simulink model "StdAnimation_Test"  (R2017b)
settings: Solver=FixedStepDiscrete  StartTime=0.0  StopTime=45  FixedStep=0.02  RelTol=1e-3  EnableMultiTasking=on
undefined symbols (not defined in the file): sigbuilder_block
settings Model: DataDictionary=Copy_of_StdAnimation_DD_New.sldd  Creator=mchawa  LastModifiedBy=oashraf
settings ConfigSet: Description=AutoGeneratedSLSFconfig
settings DataIOCC: LimitDataPoints=on  SaveOutput=off  SaveTime=off
settings OptimizationCC: DefaultParameterBehavior=Inlined  UseDivisionForNetSlopeComputation=on  DefaultUnderspecifiedDataType=single  PassReuseOutputArgsAs=Individual arguments  LifeSpan=Inf  SimCompilerOptimization=on
settings DebuggingCC: ConsistencyChecking=warning  SignalInfNanChecking=error  SignalRangeChecking=error  ReadBeforeWriteMsg=EnableAllAsError  WriteAfterWriteMsg=EnableAllAsError  WriteAfterReadMsg=EnableAllAsError  AlgebraicLoopMsg=error  ArtificialAlgebraicLoopMsg=error  SaveWithDisabledLinksMsg=error  SaveWithParameterizedLinksMsg=error  SignalResolutionControl=TryResolveAllWithWarning  BlockPriorityViolationMsg=error  MinStepSizeMsg=error  SolverPrmCheckMsg=error  InheritedTsInSrcMsg=error  SingleTaskRateTransMsg=error  TasksWithSamePriorityMsg=error  SigSpecEnsureSampleTimeMsg=error  CheckMatrixSingularityMsg=error  ParameterDowncastMsg=warning  ParameterUnderflowMsg=error  FixptConstUnderflowMsg=warning  FixptConstOverflowMsg=warning  FixptConstPrecisionLossMsg=warning  UnderSpecifiedDataTypeMsg=warning  UnnecessaryDatatypeConvMsg=warning  VectorMatrixConversionMsg=warning  SignalLabelMismatchMsg=warning  UnconnectedInputMsg=error  UnconnectedOutputMsg=error  UnconnectedLineMsg=error  SFcnCompatibilityMsg=warning  FrameProcessingCompatibilityMsg=warning  UniqueDataStoreMsg=error  BusObjectLabelMismatch=none  RootOutportRequireBusObject=error  AssertControl=DisableAll  AllowSymbolicDim=off  ModelReferenceVersionMismatchMessage=warning  ModelReferenceIOMismatchMessage=warning  UnknownTsInhSupMsg=error  ModelReferenceDataLoggingMessage=error  StateNameClashWarn=warning  StrictBusMsg=ErrorOnBusTreatedAsVector  NonBusSignalsTreatedAsBus=error  SFInvalidInputDataAccessInChartInitDiag=error  SFTransitionOutsideNaturalParentDiag=error  SFUnreachableExecutionPathDiag=error  SFUndirectedBroadcastEventsDiag=error  SFTransitionActionBeforeConditionDiag=error  SFTemporalDelaySmallerThanSampleTimeDiag=error  SFSelfTransitionDiag=error  SFMachineParentedDataDiag=error
settings HardwareCC: ProdBitPerPointer=32  ProdBitPerSizeT=32  ProdBitPerPtrDiffT=32  ProdLargestAtomicInteger=Long  ProdLargestAtomicFloat=Double  ProdWordSize=32  ProdLongLongMode=on  ProdHWDeviceType=NXP->Cortex-M0/M0+
settings ModelReferenceCC: EnableRefExpFcnMdlSchedulingChecks=off  ModelReferenceNumInstancesAllowed=Single  PropagateSignalLabelsOutOfModel=off
settings SFSimCC: SimUserSources="\"ANIM_int.c\""  MATLABDynamicMemAlloc=off
settings RTWCC: SystemTargetFile=ert.tlc  TemplateMakefile=ert_default_tmf  BuildConfiguration=Faster Runs  IncludeHyperlinkInReport=on  PortableWordSizes=on  CodeExecutionProfiling=on  CodeProfilingInstrumentation=on
settings RTWCC: CustomSource=|
  | "ANIM_int.c"
  | "ANIM_cfg.c"
settings CodeAppCC: IgnoreCustomStorageClasses=off  IgnoreTestpoints=on  SimulinkDataObjDesc=on  SFDataObjDesc=on  CustomSymbolStrType=$N$R$M  CustomSymbolStrFcn=$N$M$F  CustomSymbolStrBlkIO=loc_$N$M  CustomSymbolStrTmpVar=loc_$N$M  InsertBlockDesc=on  StateflowObjectComments=on  ReqsInCode=on
settings ERTTargetCC: UtilityFuncGeneration=Shared location  GenerateSampleERTMain=on  IncludeMdlTerminateFcn=off  CombineSignalStateStructs=on  SuppressErrorStatus=on  SupportAbsoluteTime=off  SupportNonFinite=off  SupportComplex=off  PurelyIntegerCode=on  RemoveResetFunc=off  ParenthesesLevel=Maximum  CastingMode=Standards  GenerateSharedConstants=off  GenerateASAP2=on  ERTCustomFileTemplate=example_file_process.tlc  EnableDataOwnership=on  DataDefinitionFile=ADBM_cfg.c  DataReferenceFile=ADBM_cfg.h  ConvertIfToSwitch=off  SuppressUnreachableDefaultCases=off  EnableSignedLeftShifts=off  EnableSignedRightShifts=off  MemSecPackage=mpt
settings ConfigComp: CovMetricSettings=we

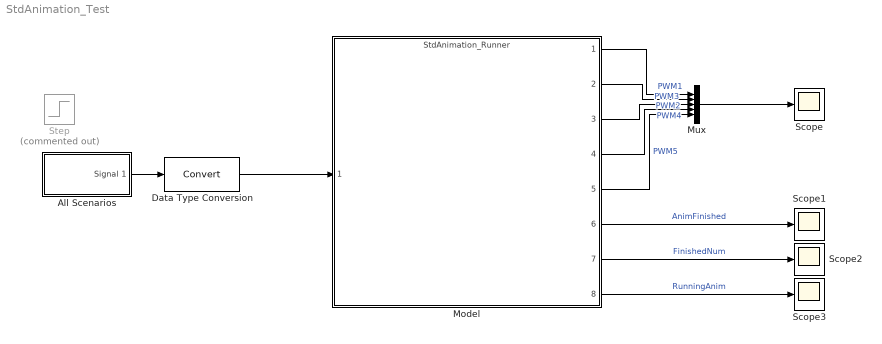
== system StdAnimation_Test ==
  All Scenarios : Subsystem  Tag=STV Subsys  LoadFcn=sigbuilder_block('load');  StartFcn=sigbuilder_block('start');  StopFcn=sigbuilder_block('stop');  ClipboardFcn=sigbuilder_block('clipboard');  mask(Sigbuilder block){tuvar=[0:10]}
      mask help: Simulink:masks:SigbuilderBlock_MD
      mask init:
      | if ~strcmp(get_param(bdroot(gcbh),'SimulationStatus'),'stopped') tuvar = sigbuilder_block('maskInit'); end
      settings: CopyFcn=sigbuilder_block('copy');  DeleteFcn=sigbuilder_block('delete');  ModelCloseFcn=sigbuilder_block('modelClose');  PreSaveFcn=sigbuilder_block('preSave');  PauseFcn=sigbuilder_block('pause');  ContinueFcn=sigbuilder_block('continue');  NameChangeFcn=sigbuilder_block('namechange');  OpenFcn=sigbuilder_block('open',[413.4 108 550.8 400.2 ]);  CloseFcn=sigbuilder_block('close');
      mask Display: plot(0, 0, 100, 100,[2, 2, 32, 32, 2], [68, 8, 8, 68, 68],[32, 2], [38, 38], [32, 19, 2],[53, 60, 44], [32, 17, 17, 2],[16, 16, 31, 31]);txt = getActiveGroup(gcbh);text(2, 100, txt,'verticalAlignment', 'top');
  Data Type Conversion : DataTypeConversion
  Model : ModelReference  ModelNameDialog=StdAnimation_Runner.slx  SimulationMode=Normal  ModelReferenceVersion=1.63
  Mux : Mux  Inputs=5
  Scope{,1..3} (4 alike) : Scope
  Step : Step  Commented=on  Time=0  After=3  SampleTime=0
  wires:
  Data Type Conversion/1 -> Model/1
  Model/3 -> Mux/3  "PWM3"
  Model/2 -> Mux/2  "PWM2"
  Model/4 -> Mux/4  "PWM4"
  Model/1 -> Mux/1  "PWM1"
  Model/5 -> Mux/5  "PWM5"
  Mux/1 -> Scope/1
  Model/6 -> Scope1/1  "AnimFinished"
  Model/8 -> Scope3/1  "RunningAnim"
  Model/7 -> Scope2/1  "FinishedNum"
  All Scenarios/1(Signal 1) -> Data Type Conversion/1

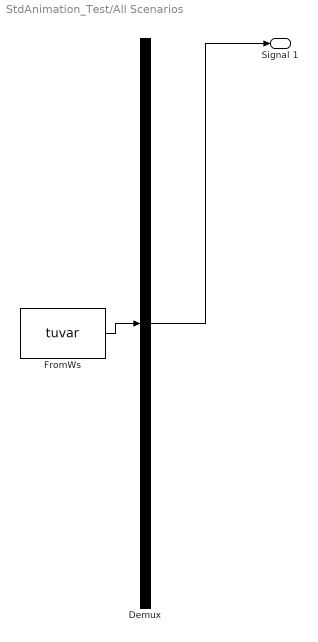
== system StdAnimation_Test/All Scenarios ==
  Demux : Demux  Tag=STV Demux  Outputs=1
      settings: DisplayOption=none
  FromWs : FromWorkspace  Tag=STV FromWs  VariableName=tuvar
      SigBuilderData=|
      | common.afterFinalStr = 'Extrapolate'
      | common.sampleTime = 0
      | dataSet.timeRange = [0 50]
      | dataSet.name = 'Group 1'
      | sbobj.Groups.Name = 'Group 1'
      | sbobj.Groups.Signals.Name = 'Signal 1'
      | sbobj.Groups.Signals.XData = [0 0.5 0.5 10.5 10.5 11 11 21 21 21.5 21.5 31.5 31.5 32 32 42 42 50]
      | sbobj.Groups.Signals.YData = [0 0 1 1 0 0 2 2 0 0 3 3 0 0 4 4 0 0]
      | sbobj.Groups.TimeRange = [0 50]
  Signal 1 : Outport  Tag=STV Outport
  wires:
  Demux/1 -> Signal 1/1
  FromWs/1 -> Demux/1
